simulink model "simActuatorPositionControl"  (R2022a)
settings: Solver=VariableStepAuto  StartTime=0.0  StopTime=10  FixedStep=0.001  MaxStep=0.01  RelTol=1e-3
InitFcn:
  | addpath('SCADA');
  | initFcn_SCADA;
model workspace (MAT data in the model file):
  WECmotionOnOff : Simulink.Parameter (value not decoded)
values from neighbouring files (symbols this model uses):
  s = scatter(X(iVar),Y(iVar),100,[color(N-i+1,:)])    [postprocess_datafiles_accum_wRV.m]
undefined symbols (not defined in the file or in its folder): g, HIL_act_A_cap, HIL_act_A_rod, HIL_H1T_kd, HIL_H1T_ki, HIL_H1T_kp, HIL_H1T_P1fBias, HIL_H1T_P1negCutIn, HIL_H1T_P1posCutIn, HIL_H1T_P2fBias, HIL_H1T_P2negCutIn, HIL_H1T_P2posCutIn, HIL_scale_sys, HIL_WECpump_A_cap, HIL_WECpump_A_rod, HIL_WECpump_ang2lin, HIL_WECpump_negativeCtrlLimit, HIL_WECpump_negativeLimit, HIL_WECpump_positiveCtrlLimit, HIL_WECpump_positiveLimit, rho, wave_phi, wave_S_w, WEC_A_rad, WEC_B_rad, WEC_dw, WEC_F_amp, WEC_h, WEC_I, WEC_I_inf, WEC_ICs, WEC_L_cm, WEC_L_flap, WEC_m, WEC_phi_e, WEC_T, WEC_W, WEC_w
libraries: fl_lib x24, sh_lib x22, nesl_utility x11, slpidlib x1, simulink x1
(part 2 of 2)

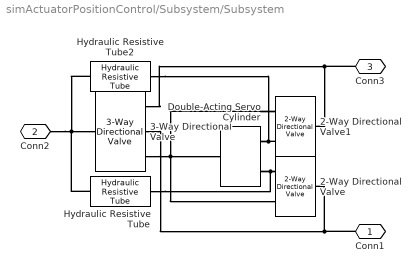
== system simActuatorPositionControl/Subsystem/Subsystem ==
  2-Way Directional Valve : sh_lib/Valves/Directional Valves/2-Way Directional Valve  mdl_type=2  area_max=0.5e-4 m^2  opening_max=0.005 m  opening_tab=[-0.5, 0.135, 0.14, 0.5] in  area_tab=[4.5239e-04, 4.5239e-04, 0, 0] in^2  pressure_tab=[-10000000, -5000000, -2000000, 2000000, 5000000, 10000000] Pa  flow_rate_tab=[-1e-07, -7.0711e-08, -4.4721e-08, 4.4721e-08, 7.0711e-08, 1e-07; -2.0352e-05, -1.4391e-05, -9.1017e-06, 9.1017e-06, 1.4391e-05, 2.0352e-05; -.0040736, -.0028805, -.0018218, .0018218, .0028805, .0040736; -.011438, -.0080879, -.0051152, .0051152, .0080879, .011438; -.034356, -.024293, -.015364, .015364, .024293, .034356] m^3/s  interp_method=1  extrap_method=1  C_d=0.7  x_0=0 in  A_leak=1e-12 m^2  lam_spec=1  B_lam=0.999  Re_cr=12
      settings: SourceProductBaseCode=SH  InternalSimscapePortConfiguration="{\"Bottom\":[],\"Left\":[{\"id\":\"S\",\"label\":\"S\",\"type\":\"input\"},{\"id\":\"A\",\"label\":\"A\",\"type\":\"foundation.hydraulic.hydraulic\"}],\"Right\":[{\"id\":\"B\",\"label\":\"B\",\"type\":\"foundation.hydraulic.hydraulic\"}],\"Top\":[]}"
  2-Way Directional Valve1 : sh_lib/Valves/Directional Valves/2-Way Directional Valve  mdl_type=2  area_max=0.5e-4 m^2  opening_max=0.005 m  opening_tab=-1*[-0.5, 0.135, 0.14, 0.5] m  area_tab=[4.5239e-04, 4.5239e-04, 0, 0] m^2  pressure_tab=[-10000000, -5000000, -2000000, 2000000, 5000000, 10000000] Pa  flow_rate_tab=[-1e-07, -7.0711e-08, -4.4721e-08, 4.4721e-08, 7.0711e-08, 1e-07; -2.0352e-05, -1.4391e-05, -9.1017e-06, 9.1017e-06, 1.4391e-05, 2.0352e-05; -.0040736, -.0028805, -.0018218, .0018218, .0028805, .0040736; -.011438, -.0080879, -.0051152, .0051152, .0080879, .011438; -.034356, -.024293, -.015364, .015364, .024293, .034356] m^3/s  interp_method=1  extrap_method=1  C_d=0.7  x_0=0 m  A_leak=1e-12 m^2  lam_spec=1  B_lam=0.999  Re_cr=12
      settings: SourceProductBaseCode=SH  InternalSimscapePortConfiguration="{\"Bottom\":[],\"Left\":[{\"id\":\"S\",\"label\":\"S\",\"type\":\"input\"},{\"id\":\"A\",\"label\":\"A\",\"type\":\"foundation.hydraulic.hydraulic\"}],\"Right\":[{\"id\":\"B\",\"label\":\"B\",\"type\":\"foundation.hydraulic.hydraulic\"}],\"Top\":[]}"
  3-Way Directional Valve : sh_lib/Valves/Directional Valves/3-Way Directional Valve  area_spec=sh.valves.directional_valves.enum.area_spec.identical  mdl_type_identical=sh.valves.directional_valves.enum.mdl_type.linear  mdl_type_different=sh.valves.directional_valves.enum.mdl_type.linear  interp_method_identical=sh.valves.directional_valves.enum.interp_method.linear  interp_method_different=sh.valves.directional_valves.enum.interp_method.linear  extrap_method_identical=sh.valves.directional_valves.enum.extrap_method.linear  extrap_method_different=sh.valves.directional_valves.enum.extrap_method.linear  A_leak=3e-7 m^2  C_d=0.7  lam_spec=sh.valves.directional_valves.enum.lam_spec.pressure_ratio  B_lam=0.999  Re_cr=12  opening_max=0.339 in  area_max=3.04e-4 m^2  opening_max_P_A=0.005 m  area_max_P_A=0.5e-4 m^2  opening_max_A_T=0.005 m  area_max_A_T=0.5e-4 m^2  opening_area_tab=[-.002, 0, .002, .005, .015] m  area_tab=[1e-09, 2.0352e-07, 4.0736e-05, .00011438, .00034356] m^2  opening_flow_rate_tab=[-.002, 0, .002, .005, .015] m  pressure_tab=[-10000000, -5000000, -2000000, 2000000, 5000000, 10000000] Pa  flow_rate_tab=[-1e-07, -7.0711e-08, -4.4721e-08, 4.4721e-08, 7.0711e-08, 1e-07; -2.0352e-05, -1.4391e-05, -9.1017e-06, 9.1017e-06, 1.4391e-05, 2.0352e-05; -.0040736, -.0028805, -.0018218, .0018218, .0028805, .0040736; -.011438, -.0080879, -.0051152, .0051152, .0080879, .011438; -.034356, -.024293, -.015364, .015364, .024293, .034356] m^3/s  opening_area_tab_P_A=[-.002, 0, .002, .005, .015] m  area_tab_P_A=[1e-09, 2.0352e-07, 4.0736e-05, .00011438, .00034356] m^2  opening_flow_rate_tab_P_A=[-.002, 0, .002, .005, .015] m  pressure_tab_P_A=[-10000000, -5000000, -2000000, 2000000, 5000000, 10000000] Pa  flow_rate_tab_P_A=[-1e-07, -7.0711e-08, -4.4721e-08, 4.4721e-08, 7.0711e-08, 1e-07; -2.0352e-05, -1.4391e-05, -9.1017e-06, 9.1017e-06, 1.4391e-05, 2.0352e-05; -.0040736, -.0028805, -.0018218, .0018218, .0028805, .0040736; -.011438, -.0080879, -.0051152, .0051152, .0080879, .011438; -.034356, -.024293, -.015364, .015364, .024293, .034356] m^3/s  opening_area_tab_A_T=[-.002, 0, .002, .005, .015] m  area_tab_A_T=[1e-09, 2.0352e-07, 4.0736e-05, .00011438, .00034356] m^2  opening_flow_rate_tab_A_T=[-.002, 0, .002, .005, .015] m  pressure_tab_A_T=[-10000000, -5000000, -2000000, 2000000, 5000000, 10000000] Pa  flow_rate_tab_A_T=[-1e-07, -7.0711e-08, -4.4721e-08, 4.4721e-08, 7.0711e-08, 1e-07; -2.0352e-05, -1.4391e-05, -9.1017e-06, 9.1017e-06, 1.4391e-05, 2.0352e-05; -.0040736, -.0028805, -.0018218, .0018218, .0028805, .0040736; -.011438, -.0080879, -.0051152, .0051152, .0080879, .011438; -.034356, -.024293, -.015364, .015364, .024293, .034356] m^3/s  x_0_P=0.027 in  x_0_T=0.027 in
      settings: SourceProductBaseCode=SH  InternalSimscapePortConfiguration="{\"Bottom\":[],\"Left\":[{\"id\":\"A\",\"label\":\"A\",\"type\":\"foundation.hydraulic.hydraulic\"}],\"Right\":[{\"id\":\"S\",\"label\":\"S\",\"type\":\"input\"},{\"id\":\"P\",\"label\":\"P\",\"type\":\"foundation.hydraulic.hydraulic\"},{\"id\":\"T\",\"label\":\"T\",\"type\":\"foundation.hydraulic.hydraulic\"}],\"Top\":[]}"
  Double-Acting Servo Cylinder : sh_lib/Valves/Valve Actuators/Double-Acting Servo Cylinder  piston_area=0.3468 in^2  stroke=0.339 cm  spring_rate=1 N/m  damping=1 N*s/m  stop_coefficient=1e12 N*s/m^2
      settings: SourceProductBaseCode=SH  InternalSimscapePortConfiguration="{\"Bottom\":[],\"Left\":[{\"id\":\"A\",\"label\":\"A\",\"type\":\"foundation.hydraulic.hydraulic\"},{\"id\":\"B\",\"label\":\"B\",\"type\":\"foundation.hydraulic.hydraulic\"}],\"Right\":[{\"id\":\"P\",\"label\":\"P\",\"type\":\"output\"}],\"Top\":[]}"
  Hydraulic Resistive Tube : fl_lib/Hydraulic/Hydraulic Elements/Hydraulic Resistive Tube  cs_type=1  d_in=0.012 in  area=1e-4 m^2  D_h=1.12e-2 m  s_factor=64  length=0.0513 in  length_ad=1 m  roughness=15e-6 m  Re_lam=2000  Re_turb=4000  q_specify=off  q_priority=None  q=1e-3 m^3/s  q_nominal_specify=off  q_nominal_unit=m^3/s  q_nominal_value=1  p_specify=off  p_priority=None  p=0 Pa  p_nominal_specify=off  p_nominal_unit=Pa  p_nominal_value=1
      settings: SourceProductBaseCode=PW,SS,VE  InternalSimscapePortConfiguration="{\"Bottom\":[],\"Left\":[{\"id\":\"A\",\"label\":\"A\",\"type\":\"foundation.hydraulic.hydraulic\"}],\"Right\":[{\"id\":\"B\",\"label\":\"B\",\"type\":\"foundation.hydraulic.hydraulic\"}],\"Top\":[]}"
  Hydraulic Resistive Tube2 : fl_lib/Hydraulic/Hydraulic Elements/Hydraulic Resistive Tube  cs_type=1  d_in=0.012 in  area=1e-4 m^2  D_h=1.12e-2 m  s_factor=64  length=0.0513 in  length_ad=1 m  roughness=15e-6 m  Re_lam=2000  Re_turb=4000  q_specify=off  q_priority=None  q=1e-3 m^3/s  q_nominal_specify=off  q_nominal_unit=m^3/s  q_nominal_value=1  p_specify=off  p_priority=None  p=0 Pa  p_nominal_specify=off  p_nominal_unit=Pa  p_nominal_value=1
      settings: SourceProductBaseCode=PW,SS,VE  InternalSimscapePortConfiguration="{\"Bottom\":[],\"Left\":[{\"id\":\"A\",\"label\":\"A\",\"type\":\"foundation.hydraulic.hydraulic\"}],\"Right\":[{\"id\":\"B\",\"label\":\"B\",\"type\":\"foundation.hydraulic.hydraulic\"}],\"Top\":[]}"
  Conn1 : PMIOPort  Side=Right
  Conn2 : PMIOPort  Port=2  Side=Left
  Conn3 : PMIOPort  Port=3  Side=Right
  connections:
  Conn2/RConn1 -- Hydraulic Resistive Tube2/LConn1 -- Hydraulic Resistive Tube/LConn1 -- 3-Way Directional Valve/LConn1
  3-Way Directional Valve/RConn1 -- 2-Way Directional Valve1/LConn1 -- Double-Acting Servo Cylinder/RConn1 -- 2-Way Directional Valve/LConn1
  Hydraulic Resistive Tube/RConn1 -- 2-Way Directional Valve/LConn2 -- Double-Acting Servo Cylinder/LConn1
  Hydraulic Resistive Tube2/RConn1 -- Double-Acting Servo Cylinder/LConn2 -- 2-Way Directional Valve1/LConn2
  3-Way Directional Valve/RConn2 -- Conn1/RConn1 -- 2-Way Directional Valve/RConn1
  3-Way Directional Valve/RConn3 -- Conn3/RConn1 -- 2-Way Directional Valve1/RConn1

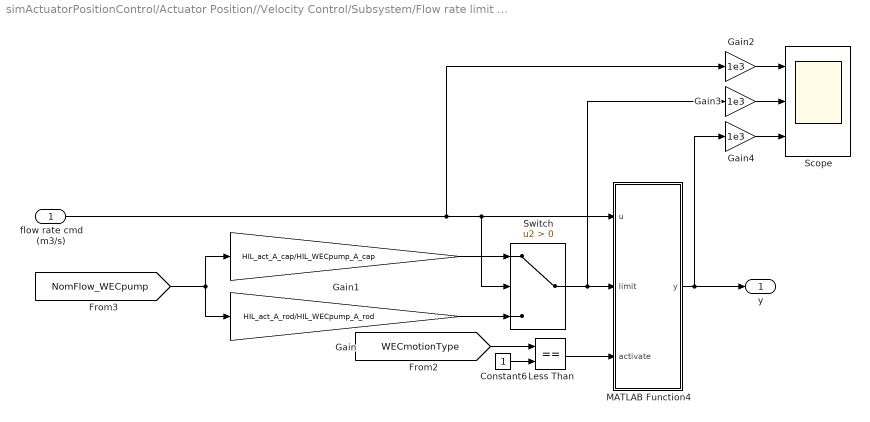
== system simActuatorPositionControl/Actuator Position//Velocity Control/Subsystem/Flow rate limit for position control ==
  flow rate cmd (m3/s) : Inport
  Constant6 : Constant
  Gain : Gain  Gain=HIL_act_A_rod/HIL_WECpump_A_rod
  Gain1 : Gain  Gain=HIL_act_A_cap/HIL_WECpump_A_cap
  Gain2 : Gain  Gain=1e3
  Gain3 : Gain  Gain=1e3
  Gain4 : Gain  Gain=1e3
  Less Than : RelationalOperator  Operator===  OutDataTypeStr=boolean  RndMeth=Simplest  InputSameDT=off
  MATLAB Function4 : MATLAB Function  TreatAsAtomicUnit=on
  Scope : Scope  NumInputPorts=3
  Switch : Switch  Criteria=u2 > Threshold  SaturateOnIntegerOverflow=off  InputSameDT=off
  y : Outport
  wires:
  Constant6/1 -> Less Than/2
  MATLAB Function4/1(y) -> y/1, Gain4/1
  Switch/1 -> Gain3/1, MATLAB Function4/2(limit)
  Less Than/1 -> MATLAB Function4/3(activate)
  [WECmotionType] -> Less Than/1
  Gain/1 -> Switch/3
  Gain1/1 -> Switch/1
  [NomFlow_WECpump] -> Gain1/1, Gain/1
  flow rate cmd (m3/s)/1 -> Gain2/1, Switch/2, MATLAB Function4/1(u)
  Gain2/1 -> Scope/1
  Gain3/1 -> Scope/2
  Gain4/1 -> Scope/3

== matlab function simActuatorPositionControl/WEC Simulation/Regular Waves ==
  data: t input; waveElev output; T_e output; WEC_F_amp parameter; WEC_w parameter; WEC_dw parameter; WEC_phi_e parameter; wave_S_w parameter; wave_phi parameter
function [waveElev,T_e] = fcn(t, WEC_F_amp, WEC_w, WEC_dw, WEC_phi_e, wave_S_w, wave_phi)

T_e = sum( WEC_F_amp.*sqrt(2*wave_S_w.*WEC_dw) ...
            .*sin(WEC_w*t + wave_phi + WEC_phi_e ));

waveElev = sum( sqrt(2*wave_S_w(:).*WEC_dw) ...
                .*sin(WEC_w(:)*t + wave_phi(:)) );

== matlab function simActuatorPositionControl/Actuator Position//Velocity Control/Subsystem/Flow rate limit for position control/MATLAB Function4 ==
  data: u input; y output; limit input; activate input
function y = fcn(u,limit,activate)
y = u ...
    + (sign(u)*limit - u) * (abs(u) >= limit) * activate;

== matlab function simActuatorPositionControl/Prescribed Motion/Prescribed Wave-like Motion/Wave-like motion ==
  data: t input; pos output; meanFlow input; w input; WECmotionType input; HIL_WECpump_A_cap parameter; HIL_WECpump_A_rod parameter
function pos = fcn(t,meanFlow,...
                w,WECmotionType,HIL_WECpump_A_cap, HIL_WECpump_A_rod)

% switch WECmotionType
%     case {0,1} % regular motion
        x_amp = meanFlow*pi/2/w/(HIL_WECpump_A_cap + HIL_WECpump_A_rod);
        
        pos = x_amp*sin(w*t);

%     case 1 % irregular motion
%         
%         pos = sum( x_amp.*sin(w.*t + psi));

% end

== matlab function simActuatorPositionControl/Subsystem/MATLAB Function1 ==
  data: duty input; f output
function f  = fcn(duty)
posCutIn = 0.23;
negCutIn = 0.23;

f = ((duty-posCutIn)/(1-posCutIn))*(duty>posCutIn) + ...
    ((duty+negCutIn)/(1-negCutIn))*(duty<-negCutIn);
f = max(-1,min(1,f));

== matlab function simActuatorPositionControl/Actuator Position//Velocity Control/Subsystem/MATLAB Function2 ==
  data: f input; dutyMag output; dutySign output; posCutIn input; negCutIn input
function [dutyMag,dutySign] = fcn(f,posCutIn, negCutIn)
duty = ((1-posCutIn)*f + posCutIn)*(f>0) + ...
    ((1-negCutIn)*f - negCutIn)*(f<0);
duty = max(-1,min(1,duty));
dutyMag = abs(duty);
dutySign = sign(duty);

== matlab function simActuatorPositionControl/Actuator Position//Velocity Control/Subsystem/Pump displacement blend ==
  data: f input; f1 output; f2 output; HIL_H1T_P1fBias parameter; HIL_H1T_P2fBias parameter
function [f1,f2] = fcn(f,HIL_H1T_P1fBias, HIL_H1T_P2fBias)
    P1 = -HIL_H1T_P1fBias;
    P2 = HIL_H1T_P2fBias;
    
    f1 = (1/(1+P1))*(f-P1) * (f<=P1) ...
       + (2*P2/(P2-P1))*(f-P1) * ((P1 < f) & (f < P2)) ...
       + ((1-2*P2)/(1-P2)*f + 1 - (1-2*P2)/(1-P2)) * (f>=P2);
    
    f2 = ((1+2*P1)/(1+P1)*f + (1+2*P1)/(1+P1) - 1) * (f<=P1) ...
       + (2*P1/(P1-P2))*(f-P2) * ((P1 < f) & (f < P2)) ...
       + (1/(1-P2))*(f-P2) * (f>=P2);

== matlab function simActuatorPositionControl/Subsystem/Mean ==
  data: u1 input; y1 output; u2 input; y2 output; y3 output
function [y1, y2, y3] = fcn(u1,u2)
y1 = u1;
y2 = u2;
y3 = mean([u1,u2]);

== stateflow chart simActuatorPositionControl/Prescribed Motion/Constant WEC-driven Pump Flow1/State Transition Table ==
  state forward
    entry:
    direction=1;
  state reverse
    entry:
    direction=0;
  (default) -> forward
  forward -> (junction 25) [order 2] : [pos<HIL_WECpump_positiveCtrlLimit]
  (junction 25) -> forward
  forward -> reverse [order 1] : [pos>=HIL_WECpump_positiveCtrlLimit]
  reverse -> forward [order 1] : [pos<=HIL_WECpump_negativeCtrlLimit]
  reverse -> (junction 29) [order 2] : [pos>HIL_WECpump_negativeCtrlLimit]
  (junction 29) -> reverse
  data: pos input; direction output; HIL_WECpump_positiveCtrlLimit parameter; HIL_WECpump_negativeCtrlLimit parameter

== matlab function simActuatorPositionControl/Actuator Position//Velocity Control/Subsystem/MATLAB Function1 ==
  data: speed_rpm input; maxFlow_m3perSec output; numPumps input; HIL_H1T_D parameter
function maxFlow_m3perSec = fcn(speed_rpm,numPumps,HIL_H1T_D)
eff_vol = 0.92;
displacement = HIL_H1T_D*(0.01)^3; % [cc/rev -> m^3/rev]
maxFlow_m3perSec = numPumps*eff_vol*speed_rpm/60*displacement;

== matlab function simActuatorPositionControl/Actuator Position//Velocity Control/Subsystem/MATLAB Function ==
  data: f input; dutyMag output; dutySign output; posCutIn input; negCutIn input
function [dutyMag,dutySign] = fcn(f,posCutIn, negCutIn)
duty = ((1-posCutIn)*f + posCutIn)*(f>0) + ...
    ((1-negCutIn)*f - negCutIn)*(f<0);
duty = max(-1,min(1,duty));
dutyMag = abs(duty);
dutySign = sign(duty);

== matlab function simActuatorPositionControl/Actuator Position//Velocity Control/Subsystem/FF flowrate ==
  data: vel input; flowrate output; HIL_act_A_cap parameter; HIL_act_A_rod parameter
function flowrate = fcn(vel,HIL_act_A_cap,HIL_act_A_rod)
flowrate = vel* ...
           (HIL_act_A_cap*(vel>=0) + ...
            HIL_act_A_rod*(vel<0));

== matlab function simActuatorPositionControl/Subsystem/MATLAB Function ==
  data: duty input; f output
function f  = fcn(duty)
posCutIn = 0.23;
negCutIn = 0.23;

f = ((duty-posCutIn)/(1-posCutIn))*(duty>posCutIn) + ...
    ((duty+negCutIn)/(1-negCutIn))*(duty<-negCutIn);
f = max(-1,min(1,f));

== matlab function simActuatorPositionControl/WEC Simulation/Irregular Waves ==
  data: t input; waveElev output; T_e output; WEC_F_amp parameter; WEC_w parameter; WEC_dw parameter; WEC_phi_e parameter; wave_S_w parameter; wave_phi parameter
function [waveElev,T_e] = fcn(t, WEC_F_amp, WEC_w, WEC_dw, WEC_phi_e, wave_S_w, wave_phi)

T_e = sum( WEC_F_amp.*sqrt(2*wave_S_w.*WEC_dw) ...
            .*sin(WEC_w*t + wave_phi + WEC_phi_e ));

waveElev = sum( sqrt(2*wave_S_w(:).*WEC_dw) ...
                .*sin(WEC_w(:)*t + wave_phi(:)) );

== matlab function simActuatorPositionControl/WEC Simulation/Hydrostatic force ==
  data: pos input; T_h output; waveElev input; WEC_L_flap parameter; WEC_h parameter; WEC_T parameter; WEC_W parameter; rho parameter; g parameter; WEC_L_cm parameter; WEC_m parameter
function T_h = fcn(pos,waveElev,...
                    WEC_L_flap,WEC_h,WEC_T,WEC_W,rho, g, WEC_L_cm, WEC_m)
%% Determine buoyant torque from submerged volume

% Height of top edge of flap from hinge
h_top = WEC_L_flap*cos(pos);

% Length of submerged part of plate (by centerline) centroids 
% from thin plate assumption
L_sub = (h_top > WEC_h+waveElev)*(WEC_h+waveElev)/cos(pos) + ...
    (h_top <= WEC_h+waveElev)*WEC_L_flap; 

% Calculate the centroid of the buoyant force, position perpendicular to
% gravity
centroid_x = L_sub/2*sin(pos);

% calculate bouyant torque
T_buoy = WEC_T*L_sub*WEC_W*rho*g*centroid_x;

%% Determine torque due to off center weight
% Calculate position of the center of mass of the flap, perpendicular to
% gravity
cm_x = WEC_L_cm*sin(pos);

% calculate torque due to weight
T_weight = WEC_m*g*cm_x;

%% Determine total effective torque
T_h = T_buoy - T_weight;
